simulink model "fig7_73"  (Simulink 6.1)
settings: Solver=ode23  StartTime=0.0  StopTime=300.0  RelTol=1e-6
settings Model: LastModifiedBy=abbas  ExtModeTrigMode=oneshot  ExtModeArmWhenConnect=off
settings DataIOCC: LimitDataPoints=off
settings OptimizationCC: BlockReduction=off  BooleanDataType=off
settings HardwareCC: TargetUnknown=on
settings STFCustomTargetCC: TargetFcnLib=ansi_tfl_tmw.mat  GenFloatMathFcnCalls=ANSI_C  ModelReferenceCompliant=off  SystemTargetFile=grt.tlc

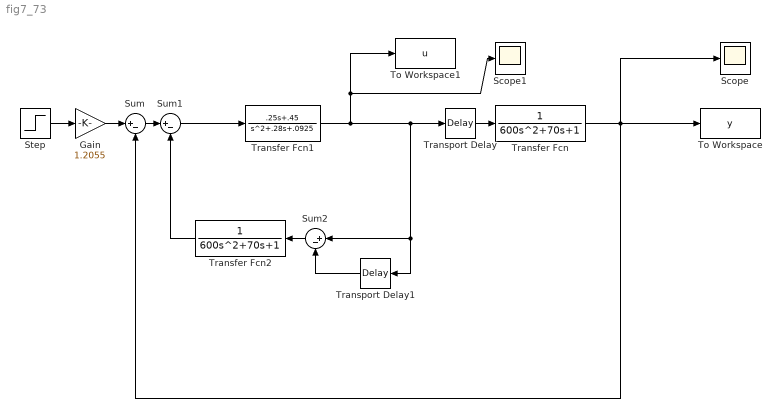
== system fig7_73 ==
  Gain : Gain  Gain=1.2055  SaturateOnIntegerOverflow=on
  Scope : Scope
  Scope1 : Scope
  Step : Step  SampleTime=0
  Sum : Sum  Inputs=|+-  SaturateOnIntegerOverflow=on  InputSameDT=on
  Sum1 : Sum  Inputs=|+-  SaturateOnIntegerOverflow=on  InputSameDT=on
  Sum2 : Sum  Orientation=left  Inputs=|+-  SaturateOnIntegerOverflow=on  InputSameDT=on
  To Workspace : ToWorkspace  VariableName=y  SampleTime=-1  SaveFormat=Array
  To Workspace1 : ToWorkspace  VariableName=u  SampleTime=-1  SaveFormat=Array
  Transfer Fcn : TransferFcn  Denominator=[600 70 1]
  Transfer Fcn1 : TransferFcn  Numerator="[.25  .45]"  Denominator=[1 .28 .0925]
  Transfer Fcn2 : TransferFcn  Orientation=left  Denominator=[600 70 1]
  Transport Delay : TransportDelay  DelayTime=5
  Transport Delay1 : TransportDelay  Orientation=left  DelayTime=5
  wires:
  Transport Delay/1 -> Transfer Fcn/1
  Transfer Fcn/1 -> To Workspace/1, Scope/1, Sum/2
  Sum1/1 -> Transfer Fcn1/1
  Sum/1 -> Sum1/1
  Transfer Fcn2/1 -> Sum1/2
  Sum2/1 -> Transfer Fcn2/1
  Transport Delay1/1 -> Sum2/2
  Transfer Fcn1/1 -> Transport Delay/1, Transport Delay1/1, Sum2/1, To Workspace1/1, Scope1/1
  Step/1 -> Gain/1
  Gain/1 -> Sum/1
